simulink model "system_closed_open"  (R2022b)
settings: Solver=VariableStepAuto  StartTime=0.0  StopTime=10.0  MaxStep=1e-3  RelTol=1e-3
settings Model: Creator=Dell  LastModifiedBy=Dell

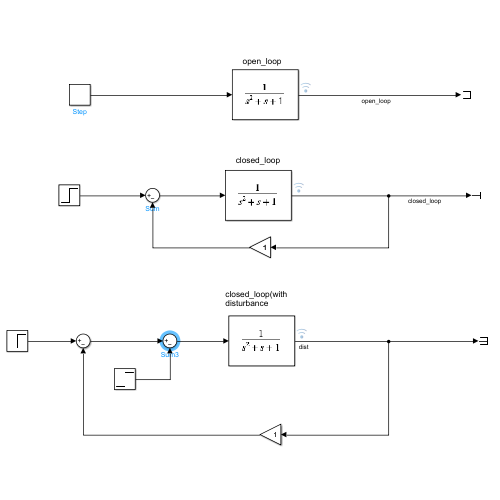
[thumbnail: Simulink's stored preview of the top-level diagram]
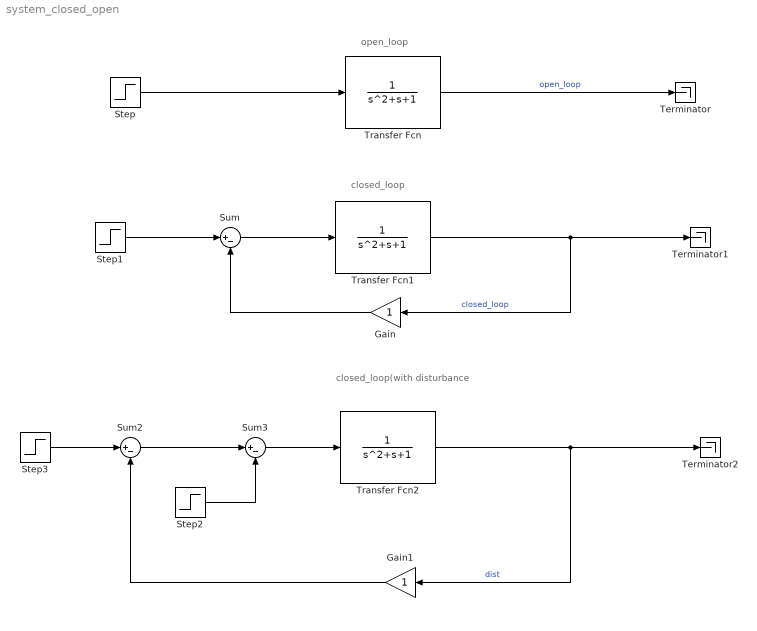
== system system_closed_open ==
  note: open_loop
  note: closed_loop
  note: closed_loop(with disturbance
  Gain : Gain
  Gain1 : Gain
  Step : Step  SampleTime=0
  Step1 : Step  SampleTime=0
  Step2 : Step  Time=4  After=0.2  SampleTime=0
  Step3 : Step  SampleTime=0
  Sum : Sum  Inputs=|+-
  Sum2 : Sum  Inputs=|+-
  Sum3 : Sum  Inputs=|+-
  Terminator : Terminator
  Terminator1 : Terminator
  Terminator2 : Terminator
  Transfer Fcn : TransferFcn  Denominator=[1 1 1]
  Transfer Fcn1 : TransferFcn  Denominator=[1 1 1]
  Transfer Fcn2 : TransferFcn  Denominator=[1 1 1]
  wires:
  Step/1 -> Transfer Fcn/1
  Transfer Fcn/1 -> Terminator/1  "open_loop"
  Transfer Fcn1/1 -> Terminator1/1, Gain/1  "closed_loop"
  Step1/1 -> Sum/1
  Gain/1 -> Sum/2
  Sum/1 -> Transfer Fcn1/1
  Sum3/1 -> Transfer Fcn2/1
  Sum2/1 -> Sum3/1
  Gain1/1 -> Sum2/2
  Step3/1 -> Sum2/1
  Transfer Fcn2/1 -> Terminator2/1, Gain1/1  "dist"
  Step2/1 -> Sum3/2
